simulink model "HIL_Testing_SW"  (Simulink 7.5)
settings: Solver=ode1  StartTime=0.0  StopTime=Inf  FixedStep=0.001  RelTol=1e-3
PostLoadFcn:
  | , if any(exist('dsrtsu_mdlpostloadfcn', 'file') == [2, 3, 6]), try dsrtsu_mdlpostloadfcn('Execute', bdroot); catch fprintf('Error in PostLoadFcn (dsrtsu_mdlpostloadfcn) for model "%s":\n %s\n', bdroot, lasterr); end, end,
undefined symbols (not defined in the file): CeBSER_Cnt_NumTempAxisPts, ChargeCord, ChargeCord_Control, ChargeToSOCCurr, ChrgCurrLim, CrntSens1Fine, CS_SOCSetPt, CyclerMaxChrgPwr, CyclerMaxDschrgPwr, deltaAhr, Drive_1, Drive_10, Drive_11, Drive_12, Drive_13, Drive_14, Drive_15, Drive_16, Drive_17, Drive_18, Drive_19, Drive_2, Drive_20, Drive_21, Drive_22, Drive_23, Drive_24, Drive_25, Drive_26, Drive_27, Drive_28, Drive_29, Drive_3, Drive_30, Drive_31, Drive_32, Drive_33, Drive_34, Drive_35, Drive_36, Drive_37, Drive_38, Drive_39, Drive_4, Drive_40, Drive_41, Drive_42, Drive_43, Drive_44, Drive_45, Drive_46, Drive_47, Drive_48, Drive_49, Drive_5, Drive_50, Drive_51, Drive_6, Drive_7, Drive_8 ... (+50)
libraries: simulink x129, rtican x50, rti2211sailib x5, rti2211serlib x5, rti2202miolib x3
(part 20 of 23)

== system HIL_Testing_SW/TX/Chiller/ChillerCmndTxDecision/ChillerRxProcessing/ReadChillerSP/RxReadChillerSP7Bytes ==
  Action Port : ActionPort  ActionType=then
  ASCIILUTable : Lookup  InputValues=[48,49,50,51,52,53,54,55,56,57]  Table=[0,1,2,3,4,5,6,7,8,9]  LookUpMeth=Use Input Nearest  OutDataTypeMode=single  OutDataType=fixdt(1, 16)  OutScaling=2^0  OutDataTypeStr=single  RndMeth=Nearest
  ASCIILUTable1 : Lookup  InputValues=[48,49,50,51,52,53,54,55,56,57]  Table=[0,1,2,3,4,5,6,7,8,9]  LookUpMeth=Use Input Nearest  OutDataTypeMode=single  OutDataType=fixdt(1, 16)  OutScaling=2^0  OutDataTypeStr=single  RndMeth=Nearest
  ASCIILUTable2 : Lookup  InputValues=[48,49,50,51,52,53,54,55,56,57]  Table=[0,.1,.2,.3,.4,.5,.6,.7,.8,.9]  LookUpMeth=Use Input Nearest  OutDataTypeMode=single  OutDataType=fixdt(1, 16)  OutScaling=2^0  OutDataTypeStr=single  RndMeth=Nearest
  Add : Sum  Inputs=+++  OutDataType=fixdt(1, 16)  OutScaling=2^-10
  Constant : Constant  Value=43  OutDataTypeMode=uint16  OutDataType=fixdt(1, 16)  OutScaling=2^0  OutDataTypeStr=uint16
  Constant1 : Constant  Value=10  OutDataTypeMode=single  OutDataType=fixdt(1, 16)  OutScaling=2^0  OutDataTypeStr=single
  Constant4 : Constant  Value=-1  OutDataTypeMode=single  OutDataType=fixdt(1, 16)  OutScaling=2^0  OutDataTypeStr=single
  Constant5 : Constant  OutDataTypeMode=single  OutDataType=fixdt(1, 16)  OutScaling=2^0  OutDataTypeStr=single
  Data Store Read1 : DataStoreRead  DataStoreName=RxChillerFIFO  SampleTime=-1
  Demux : Demux  Outputs=7
  Gain : Gain  ParameterDataType=fixdt(1, 16)  ParameterScaling=2^0  OutDataType=fixdt(1, 16)  OutScaling=2^0
  Product : Product  OutDataType=fixdt(1, 16)  OutScaling=2^0  RndMeth=Zero
  Product1 : Product  OutDataTypeMode=single  OutDataType=fixdt(1, 16)  OutScaling=2^0  OutDataTypeStr=single  RndMeth=Zero
  Relational Operator3 : RelationalOperator  Operator===  LogicOutDataTypeMode=boolean  LogicDataType=fixdt(0, 8)  OutDataTypeStr=boolean
  Switch : Switch  Threshold=1  OutDataType=fixdt(1, 16)  OutScaling=2^0
  Terminator2 : Terminator
  Terminator3 : Terminator
  Terminator4 : Terminator
  RxReadChillerSetPoint : Outport  OutDataType=fixdt(1, 16)  OutScaling=2^0
  wires:
  [RxByteOne] -> Relational Operator3/1
  Constant/1 -> Relational Operator3/2
  [RxByteFour] -> ASCIILUTable1/1
  Relational Operator3/1 -> Switch/2
  Constant5/1 -> Switch/1
  Constant4/1 -> Switch/3
  Switch/1 -> [Sign]
  Constant1/1 -> Product/2
  [RxByteThree] -> ASCIILUTable/1
  ASCIILUTable/1 -> Product/1
  Product/1 -> [TensNumber]
  ASCIILUTable1/1 -> [OnesNumber]
  [RxByteSix] -> ASCIILUTable2/1
  ASCIILUTable2/1 -> [TenthsNumber]
  [TensNumber] -> Add/1
  [OnesNumber] -> Add/2
  [TenthsNumber] -> Add/3
  Add/1 -> Product1/2  "AddedChillSP"
  Demux/1 -> [RxByteOne]
  Demux/2 -> Terminator2/1
  Demux/3 -> [RxByteThree]
  Demux/4 -> [RxByteFour]
  Demux/5 -> Terminator3/1
  Demux/6 -> [RxByteSix]
  Demux/7 -> Terminator4/1
  Data Store Read1/1 -> Demux/1
  [Sign] -> Product1/1
  Product1/1 -> Gain/1
  Gain/1 -> RxReadChillerSetPoint/1

== system HIL_Testing_SW/TX/Chiller/ChillerCmndTxDecision/ChillerRxProcessing/ReadChillerTemp/RxReadChillerTemp4Bytes ==
  Action Port : ActionPort  ActionType=elseif
  ASCIILUTable : Lookup  InputValues=[48,49,50,51,52,53,54,55,56,57]  Table=[0,1,2,3,4,5,6,7,8,9]  LookUpMeth=Use Input Nearest  OutDataTypeMode=single  OutDataType=fixdt(1, 16)  OutScaling=2^0  OutDataTypeStr=single  RndMeth=Nearest
  ASCIILUTable1 : Lookup  InputValues=[48,49,50,51,52,53,54,55,56,57]  Table=[0,1,2,3,4,5,6,7,8,9]  LookUpMeth=Use Input Nearest  OutDataTypeMode=single  OutDataType=fixdt(1, 16)  OutScaling=2^0  OutDataTypeStr=single  RndMeth=Nearest
  Add : Sum  Inputs=+++  OutDataType=fixdt(1, 16)  OutScaling=2^-10
  Constant : Constant  Value=43  OutDataTypeMode=uint16  OutDataType=fixdt(1, 16)  OutScaling=2^0  OutDataTypeStr=uint16
  Constant1 : Constant  Value=10  OutDataTypeMode=single  OutDataType=fixdt(1, 16)  OutScaling=2^0  OutDataTypeStr=single
  Constant2 : Constant  Value=0  OutDataTypeMode=single  OutDataType=fixdt(1, 16)  OutScaling=2^0  OutDataTypeStr=single
  Constant4 : Constant  Value=-1  OutDataTypeMode=single  OutDataType=fixdt(1, 16)  OutScaling=2^0  OutDataTypeStr=single
  Constant5 : Constant  OutDataTypeMode=single  OutDataType=fixdt(1, 16)  OutScaling=2^0  OutDataTypeStr=single
  Data Store Read1 : DataStoreRead  DataStoreName=RxChillerFIFO  SampleTime=-1
  Demux : Demux  Outputs=7
  Gain : Gain  ParameterDataType=fixdt(1, 16)  ParameterScaling=2^0  OutDataType=fixdt(1, 16)  OutScaling=2^0
  Product : Product  OutDataType=fixdt(1, 16)  OutScaling=2^0  RndMeth=Zero
  Product1 : Product  OutDataTypeMode=single  OutDataType=fixdt(1, 16)  OutScaling=2^0  OutDataTypeStr=single  RndMeth=Zero
  Relational Operator3 : RelationalOperator  Operator===  LogicOutDataTypeMode=boolean  LogicDataType=fixdt(0, 8)  OutDataTypeStr=boolean
  Switch : Switch  Threshold=1  OutDataType=fixdt(1, 16)  OutScaling=2^0
  Terminator{2..5} (4 alike) : Terminator
  RxReadChillerSetPoint : Outport  OutDataType=fixdt(1, 16)  OutScaling=2^0
  wires:
  [Sign] -> Product1/1
  Data Store Read1/1 -> Demux/1
  Demux/7 -> Terminator5/1
  Demux/6 -> Terminator4/1
  Demux/4 -> Terminator2/1
  Demux/3 -> [RxByteThree]
  Demux/2 -> [RxByteTwo]
  Demux/1 -> [RxByteOne]
  Add/1 -> Product1/2
  [TenthsNumber] -> Add/3
  [OnesNumber] -> Add/2
  [TensNumber] -> Add/1
  ASCIILUTable1/1 -> [OnesNumber]
  Product/1 -> [TensNumber]
  ASCIILUTable/1 -> Product/1
  [RxByteTwo] -> ASCIILUTable/1
  Constant1/1 -> Product/2
  Switch/1 -> [Sign]
  Constant4/1 -> Switch/3
  Constant5/1 -> Switch/1
  Relational Operator3/1 -> Switch/2
  [RxByteThree] -> ASCIILUTable1/1
  Constant/1 -> Relational Operator3/2
  [RxByteOne] -> Relational Operator3/1
  Constant2/1 -> [TenthsNumber]
  Demux/5 -> Terminator3/1
  Product1/1 -> Gain/1
  Gain/1 -> RxReadChillerSetPoint/1

== system HIL_Testing_SW/TX/Chiller/ChillerCmndTxDecision/ChillerRxProcessing/ReadChillerTemp/RxReadChillerTemp7Bytes ==
  Action Port : ActionPort  ActionType=then
  ASCIILUTable : Lookup  InputValues=[48,49,50,51,52,53,54,55,56,57]  Table=[0,1,2,3,4,5,6,7,8,9]  LookUpMeth=Use Input Nearest  OutDataTypeMode=single  OutDataType=fixdt(1, 16)  OutScaling=2^0  OutDataTypeStr=single  RndMeth=Nearest
  ASCIILUTable1 : Lookup  InputValues=[48,49,50,51,52,53,54,55,56,57]  Table=[0,1,2,3,4,5,6,7,8,9]  LookUpMeth=Use Input Nearest  OutDataTypeMode=single  OutDataType=fixdt(1, 16)  OutScaling=2^0  OutDataTypeStr=single  RndMeth=Nearest
  ASCIILUTable2 : Lookup  InputValues=[48,49,50,51,52,53,54,55,56,57]  Table=[0,.1,.2,.3,.4,.5,.6,.7,.8,.9]  LookUpMeth=Use Input Nearest  OutDataTypeMode=single  OutDataType=fixdt(1, 16)  OutScaling=2^0  OutDataTypeStr=single  RndMeth=Nearest
  Add : Sum  Inputs=+++  OutDataType=fixdt(1, 16)  OutScaling=2^-10
  Constant : Constant  Value=43  OutDataTypeMode=uint16  OutDataType=fixdt(1, 16)  OutScaling=2^0  OutDataTypeStr=uint16
  Constant1 : Constant  Value=10  OutDataTypeMode=single  OutDataType=fixdt(1, 16)  OutScaling=2^0  OutDataTypeStr=single
  Constant4 : Constant  Value=-1  OutDataTypeMode=single  OutDataType=fixdt(1, 16)  OutScaling=2^0  OutDataTypeStr=single
  Constant5 : Constant  OutDataTypeMode=single  OutDataType=fixdt(1, 16)  OutScaling=2^0  OutDataTypeStr=single
  Data Store Read1 : DataStoreRead  DataStoreName=RxChillerFIFO  SampleTime=-1
  Demux : Demux  Outputs=7
  Gain : Gain  ParameterDataType=fixdt(1, 16)  ParameterScaling=2^0  OutDataType=fixdt(1, 16)  OutScaling=2^0
  Product : Product  OutDataTypeMode=single  OutDataType=fixdt(1, 16)  OutScaling=2^0  OutDataTypeStr=single  RndMeth=Zero
  Product1 : Product  OutDataTypeMode=single  OutDataType=fixdt(1, 16)  OutScaling=2^0  OutDataTypeStr=single  RndMeth=Zero
  Relational Operator3 : RelationalOperator  Operator===  LogicOutDataTypeMode=boolean  LogicDataType=fixdt(0, 8)  OutDataTypeStr=boolean
  Switch : Switch  Threshold=1  OutDataTypeMode=single  OutDataType=fixdt(1, 16)  OutScaling=2^0  OutDataTypeStr=single
  Terminator2 : Terminator
  Terminator3 : Terminator
  Terminator4 : Terminator
  RxReadChillerSetPoint : Outport  OutDataType=fixdt(1, 16)  OutScaling=2^0
  wires:
  [RxByteOne] -> Relational Operator3/1
  Constant/1 -> Relational Operator3/2
  [RxByteFour] -> ASCIILUTable1/1
  Relational Operator3/1 -> Switch/2
  Constant5/1 -> Switch/1
  Constant4/1 -> Switch/3
  Switch/1 -> [Sign]
  Constant1/1 -> Product/2
  [RxByteThree] -> ASCIILUTable/1
  ASCIILUTable/1 -> Product/1
  Product/1 -> [TensNumber]
  ASCIILUTable1/1 -> [OnesNumber]
  [RxByteSix] -> ASCIILUTable2/1
  ASCIILUTable2/1 -> [TenthsNumber]
  [TensNumber] -> Add/1
  [OnesNumber] -> Add/2
  [TenthsNumber] -> Add/3
  Add/1 -> Product1/2  "AddedChillSP"
  [Sign] -> Product1/1
  Product1/1 -> Gain/1
  Demux/1 -> [RxByteOne]
  Demux/2 -> Terminator2/1
  Demux/3 -> [RxByteThree]
  Demux/4 -> [RxByteFour]
  Demux/5 -> Terminator3/1
  Demux/6 -> [RxByteSix]
  Demux/7 -> Terminator4/1
  Data Store Read1/1 -> Demux/1
  Gain/1 -> RxReadChillerSetPoint/1

== system HIL_Testing_SW/TX/Chiller/ChillerCmndTxDecision/ChillerRxProcessing/RxChillerByteShifter/NoShiftDaFIFO1 ==
  note: No Shift FIFO
  In1 : Inport  OutDataType=fixdt(1, 16)  OutScaling=2^0
  Action Port : ActionPort  ActionType=elseif
  Demux1 : Demux  Outputs=7
  Gain{,1..7} (8 alike) : Gain  ParameterDataType=fixdt(1, 16)  ParameterScaling=2^0  OutDataTypeMode=uint8  OutDataType=fixdt(1, 16)  OutScaling=2^0  OutDataTypeStr=uint8
  Mux : Mux  Inputs=7
  Out1 : Outport  OutDataType=fixdt(1, 16)  OutScaling=2^0
  wires:
  Mux/1 -> Gain7/1
  [RxByteOne] -> Mux/1
  [RxByteTwo] -> Mux/2
  [RxByteThree] -> Mux/3
  [RxByteFour] -> Mux/4
  [RxByteFive] -> Mux/5
  [RxByteSix] -> Mux/6
  [RxByteSeven] -> Mux/7
  Demux1/1 -> Gain/1
  Demux1/2 -> Gain1/1
  Demux1/3 -> Gain2/1
  Demux1/4 -> Gain3/1
  Demux1/5 -> Gain4/1
  Demux1/6 -> Gain5/1
  Demux1/7 -> Gain6/1
  Gain/1 -> [RxByteOne]
  Gain1/1 -> [RxByteTwo]
  Gain2/1 -> [RxByteThree]
  Gain3/1 -> [RxByteFour]
  Gain4/1 -> [RxByteFive]
  Gain5/1 -> [RxByteSix]
  Gain6/1 -> [RxByteSeven]
  In1/1 -> Demux1/1
  Gain7/1 -> Out1/1

== system HIL_Testing_SW/TX/Chiller/ChillerCmndTxDecision/ChillerRxProcessing/RxChillerByteShifter/NoShiftDaFIFO2 ==
  note: No Shift FIFO
  In1 : Inport  OutDataType=fixdt(1, 16)  OutScaling=2^0
  Action Port : ActionPort  ActionType=else
  Demux1 : Demux  Outputs=7
  Gain{,1..7} (8 alike) : Gain  ParameterDataType=fixdt(1, 16)  ParameterScaling=2^0  OutDataTypeMode=uint8  OutDataType=fixdt(1, 16)  OutScaling=2^0  OutDataTypeStr=uint8
  Mux : Mux  Inputs=7
  Out1 : Outport  OutDataType=fixdt(1, 16)  OutScaling=2^0
  wires:
  Gain7/1 -> Out1/1
  In1/1 -> Demux1/1
  Gain6/1 -> [RxByteSeven]
  Gain5/1 -> [RxByteSix]
  Gain4/1 -> [RxByteFive]
  Gain3/1 -> [RxByteFour]
  Gain2/1 -> [RxByteThree]
  Gain1/1 -> [RxByteTwo]
  Gain/1 -> [RxByteOne]
  Demux1/7 -> Gain6/1
  Demux1/6 -> Gain5/1
  Demux1/5 -> Gain4/1
  Demux1/4 -> Gain3/1
  Demux1/3 -> Gain2/1
  Demux1/2 -> Gain1/1
  Demux1/1 -> Gain/1
  [RxByteSeven] -> Mux/7
  [RxByteSix] -> Mux/6
  [RxByteFive] -> Mux/5
  [RxByteFour] -> Mux/4
  [RxByteThree] -> Mux/3
  [RxByteTwo] -> Mux/2
  [RxByteOne] -> Mux/1
  Mux/1 -> Gain7/1

== system HIL_Testing_SW/TX/Chiller/ChillerCmndTxDecision/ChillerRxProcessing/RxChillerByteShifter/PositiveResponseNoShift ==
  note: No Shift FIFO Right
  In1 : Inport  OutDataType=fixdt(1, 16)  OutScaling=2^0
  Action Port : ActionPort  ActionType=then
  Demux1 : Demux  Outputs=7
  Gain{,1..7} (8 alike) : Gain  ParameterDataType=fixdt(1, 16)  ParameterScaling=2^0  OutDataTypeMode=uint8  OutDataType=fixdt(1, 16)  OutScaling=2^0  OutDataTypeStr=uint8
  Mux : Mux  Inputs=7
  Out1 : Outport  OutDataType=fixdt(1, 16)  OutScaling=2^0
  wires:
  Mux/1 -> Gain7/1
  Demux1/1 -> Gain/1
  Demux1/2 -> Gain1/1
  Demux1/3 -> Gain2/1
  Demux1/4 -> Gain3/1
  Demux1/5 -> Gain4/1
  Demux1/6 -> Gain5/1
  Demux1/7 -> Gain6/1
  Gain/1 -> [RxByteOne]
  Gain1/1 -> [RxByteTwo]
  Gain2/1 -> [RxByteThree]
  Gain3/1 -> [RxByteFour]
  Gain4/1 -> [RxByteFive]
  Gain5/1 -> [RxByteSix]
  Gain6/1 -> [RxByteSeven]
  In1/1 -> Demux1/1
  Gain7/1 -> Out1/1
  [RxByteSeven] -> Mux/7
  [RxByteSix] -> Mux/6
  [RxByteFive] -> Mux/5
  [RxByteFour] -> Mux/4
  [RxByteThree] -> Mux/3
  [RxByteTwo] -> Mux/2
  [RxByteOne] -> Mux/1

== system HIL_Testing_SW/TX/Chiller/ChillerCmndTxDecision/ChillerRxProcessing/RxChillerByteShifter/ShiftFIFO_FiveRight ==
  note: Shift FIFO Five Right
  In1 : Inport  OutDataType=fixdt(1, 16)  OutScaling=2^0
  Action Port : ActionPort  ActionType=elseif
  Demux : Demux  Outputs=7
  Gain{,1..7} (8 alike) : Gain  ParameterDataType=fixdt(1, 16)  ParameterScaling=2^0  OutDataTypeMode=uint8  OutDataType=fixdt(1, 16)  OutScaling=2^0  OutDataTypeStr=uint8
  Mux : Mux  Inputs=7
  Out1 : Outport  OutDataType=fixdt(1, 16)  OutScaling=2^0
  wires:
  Mux/1 -> Gain7/1
  Demux/1 -> Gain/1
  Demux/2 -> Gain1/1
  Demux/3 -> Gain2/1
  Demux/4 -> Gain3/1
  Demux/5 -> Gain4/1
  Demux/6 -> Gain5/1
  Demux/7 -> Gain6/1
  In1/1 -> Demux/1
  Gain/1 -> [RxByteOne]
  Gain1/1 -> [RxByteTwo]
  Gain2/1 -> [RxByteThree]
  Gain3/1 -> [RxByteFour]
  Gain4/1 -> [RxByteFive]
  Gain5/1 -> [RxByteSix]
  Gain6/1 -> [RxByteSeven]
  Gain7/1 -> Out1/1
  [RxByteOne] -> Mux/6
  [RxByteSeven] -> Mux/5
  [RxByteSix] -> Mux/4
  [RxByteFive] -> Mux/3
  [RxByteFour] -> Mux/2
  [RxByteThree] -> Mux/1
  [RxByteTwo] -> Mux/7

== system HIL_Testing_SW/TX/Chiller/ChillerCmndTxDecision/ChillerRxProcessing/RxChillerByteShifter/ShiftFIFO_FourRight ==
  note: Shift FIFO Four Right
  In1 : Inport  OutDataType=fixdt(1, 16)  OutScaling=2^0
  Action Port : ActionPort  ActionType=elseif
  Demux1 : Demux  Outputs=7
  Gain{,1..7} (8 alike) : Gain  ParameterDataType=fixdt(1, 16)  ParameterScaling=2^0  OutDataTypeMode=uint8  OutDataType=fixdt(1, 16)  OutScaling=2^0  OutDataTypeStr=uint8
  Mux : Mux  Inputs=7
  Out1 : Outport  OutDataType=fixdt(1, 16)  OutScaling=2^0
  wires:
  Mux/1 -> Gain7/1
  [RxByteThree] -> Mux/7
  [RxByteTwo] -> Mux/6
  [RxByteOne] -> Mux/5
  [RxByteSeven] -> Mux/4
  [RxByteSix] -> Mux/3
  [RxByteFour] -> Mux/1
  [RxByteFive] -> Mux/2
  Demux1/1 -> Gain/1
  Demux1/2 -> Gain1/1
  Demux1/3 -> Gain2/1
  Demux1/4 -> Gain3/1
  Demux1/5 -> Gain4/1
  Demux1/6 -> Gain5/1
  Demux1/7 -> Gain6/1
  Gain/1 -> [RxByteOne]
  Gain1/1 -> [RxByteTwo]
  Gain2/1 -> [RxByteThree]
  Gain3/1 -> [RxByteFour]
  Gain4/1 -> [RxByteFive]
  Gain5/1 -> [RxByteSix]
  Gain6/1 -> [RxByteSeven]
  In1/1 -> Demux1/1
  Gain7/1 -> Out1/1

== system HIL_Testing_SW/TX/Chiller/ChillerCmndTxDecision/ChillerRxProcessing/RxChillerByteShifter/ShiftFIFO_OneRight ==
  note: Shift FIFO One Right
  In1 : Inport  OutDataType=fixdt(1, 16)  OutScaling=2^0
  Action Port : ActionPort  ActionType=elseif
  Demux1 : Demux  Outputs=7
  Gain{,1..7} (8 alike) : Gain  ParameterDataType=fixdt(1, 16)  ParameterScaling=2^0  OutDataTypeMode=uint8  OutDataType=fixdt(1, 16)  OutScaling=2^0  OutDataTypeStr=uint8
  Mux : Mux  Inputs=7
  Out1 : Outport  OutDataType=fixdt(1, 16)  OutScaling=2^0
  wires:
  Mux/1 -> Gain7/1
  Demux1/1 -> Gain/1
  Demux1/2 -> Gain1/1
  Demux1/3 -> Gain2/1
  Demux1/4 -> Gain3/1
  Demux1/5 -> Gain4/1
  Demux1/6 -> Gain5/1
  Demux1/7 -> Gain6/1
  Gain/1 -> [RxByteOne]
  Gain1/1 -> [RxByteTwo]
  Gain2/1 -> [RxByteThree]
  Gain3/1 -> [RxByteFour]
  Gain4/1 -> [RxByteFive]
  Gain5/1 -> [RxByteSix]
  Gain6/1 -> [RxByteSeven]
  In1/1 -> Demux1/1
  Gain7/1 -> Out1/1
  [RxByteTwo] -> Mux/3
  [RxByteThree] -> Mux/4
  [RxByteFour] -> Mux/5
  [RxByteFive] -> Mux/6
  [RxByteSix] -> Mux/7
  [RxByteOne] -> Mux/2
  [RxByteSeven] -> Mux/1

== system HIL_Testing_SW/TX/Chiller/ChillerCmndTxDecision/ChillerRxProcessing/RxChillerByteShifter/ShiftFIFO_SixRight ==
  note: Shift FIFO Six Right
  In1 : Inport  OutDataType=fixdt(1, 16)  OutScaling=2^0
  Action Port : ActionPort  ActionType=elseif
  Demux : Demux  Outputs=7
  Gain{,1..7} (8 alike) : Gain  ParameterDataType=fixdt(1, 16)  ParameterScaling=2^0  OutDataTypeMode=uint8  OutDataType=fixdt(1, 16)  OutScaling=2^0  OutDataTypeStr=uint8
  Mux : Mux  Inputs=7
  Out1 : Outport  OutDataType=fixdt(1, 16)  OutScaling=2^0
  wires:
  Demux/1 -> Gain/1
  Demux/2 -> Gain1/1
  Demux/3 -> Gain2/1
  Demux/4 -> Gain3/1
  Demux/5 -> Gain4/1
  Demux/6 -> Gain5/1
  Demux/7 -> Gain6/1
  In1/1 -> Demux/1
  Mux/1 -> Gain7/1
  Gain6/1 -> [RxByteSeven]
  Gain5/1 -> [RxByteSix]
  Gain4/1 -> [RxByteFive]
  Gain3/1 -> [RxByteFour]
  Gain2/1 -> [RxByteThree]
  Gain1/1 -> [RxByteTwo]
  Gain/1 -> [RxByteOne]
  Gain7/1 -> Out1/1
  [RxByteOne] -> Mux/7
  [RxByteSeven] -> Mux/6
  [RxByteSix] -> Mux/5
  [RxByteFive] -> Mux/4
  [RxByteFour] -> Mux/3
  [RxByteThree] -> Mux/2
  [RxByteTwo] -> Mux/1

== system HIL_Testing_SW/TX/Chiller/ChillerCmndTxDecision/ChillerRxProcessing/RxChillerByteShifter/ShiftFIFO_ThreeRight ==
  note: Shift FIFO Three Right
  In2 : Inport  OutDataType=fixdt(1, 16)  OutScaling=2^0
  Action Port : ActionPort  ActionType=elseif
  Demux2 : Demux  Outputs=7
  Gain{8..15} (8 alike) : Gain  ParameterDataType=fixdt(1, 16)  ParameterScaling=2^0  OutDataTypeMode=uint8  OutDataType=fixdt(1, 16)  OutScaling=2^0  OutDataTypeStr=uint8
  Mux1 : Mux  Inputs=7
  Out2 : Outport  OutDataType=fixdt(1, 16)  OutScaling=2^0
  wires:
  Mux1/1 -> Gain15/1
  [RxByteSix] -> Mux1/2
  [RxByteSeven] -> Mux1/3
  [RxByteOne] -> Mux1/4
  [RxByteTwo] -> Mux1/5
  [RxByteThree] -> Mux1/6
  [RxByteFour] -> Mux1/7
  [RxByteFive] -> Mux1/1
  Demux2/1 -> Gain8/1
  Demux2/2 -> Gain9/1
  Demux2/3 -> Gain10/1
  Demux2/4 -> Gain11/1
  Demux2/5 -> Gain12/1
  Demux2/6 -> Gain13/1
  Demux2/7 -> Gain14/1
  Gain8/1 -> [RxByteOne]
  Gain9/1 -> [RxByteTwo]
  Gain10/1 -> [RxByteThree]
  Gain11/1 -> [RxByteFour]
  Gain12/1 -> [RxByteFive]
  Gain13/1 -> [RxByteSix]
  Gain14/1 -> [RxByteSeven]
  In2/1 -> Demux2/1
  Gain15/1 -> Out2/1

== system HIL_Testing_SW/TX/Chiller/ChillerCmndTxDecision/ChillerRxProcessing/RxChillerByteShifter/ShiftFIFO_TwoRight ==
  note: Shift FIFO Two Right
  In1 : Inport  OutDataType=fixdt(1, 16)  OutScaling=2^0
  Action Port : ActionPort  ActionType=elseif
  Demux : Demux  Outputs=7
  Gain{,1..7} (8 alike) : Gain  ParameterDataType=fixdt(1, 16)  ParameterScaling=2^0  OutDataTypeMode=uint8  OutDataType=fixdt(1, 16)  OutScaling=2^0  OutDataTypeStr=uint8
  Mux : Mux  Inputs=7
  Out1 : Outport  OutDataType=fixdt(1, 16)  OutScaling=2^0
  wires:
  Mux/1 -> Gain7/1
  [RxByteSeven] -> Mux/2
  [RxByteOne] -> Mux/3
  [RxByteTwo] -> Mux/4
  [RxByteThree] -> Mux/5
  [RxByteFour] -> Mux/6
  [RxByteFive] -> Mux/7
  [RxByteSix] -> Mux/1
  Demux/1 -> Gain/1
  Demux/2 -> Gain1/1
  Demux/3 -> Gain2/1
  Demux/4 -> Gain3/1
  Demux/5 -> Gain4/1
  Demux/6 -> Gain5/1
  Demux/7 -> Gain6/1
  In1/1 -> Demux/1
  Gain/1 -> [RxByteOne]
  Gain1/1 -> [RxByteTwo]
  Gain2/1 -> [RxByteThree]
  Gain3/1 -> [RxByteFour]
  Gain4/1 -> [RxByteFive]
  Gain5/1 -> [RxByteSix]
  Gain6/1 -> [RxByteSeven]
  Gain7/1 -> Out1/1

== system HIL_Testing_SW/TX/Chiller/ChillerCmndTxDecision/ChillerRxProcessing/RxChillerByteShifter/SwapByte1And2 ==
  note: SwapByte1And2
  In1 : Inport  OutDataType=fixdt(1, 16)  OutScaling=2^0
  Action Port : ActionPort  ActionType=elseif
  Demux1 : Demux  Outputs=7
  Gain{,1..7} (8 alike) : Gain  ParameterDataType=fixdt(1, 16)  ParameterScaling=2^0  OutDataTypeMode=uint8  OutDataType=fixdt(1, 16)  OutScaling=2^0  OutDataTypeStr=uint8
  Mux : Mux  Inputs=7
  Out1 : Outport  OutDataType=fixdt(1, 16)  OutScaling=2^0
  wires:
  [RxByteThree] -> Mux/3
  [RxByteFour] -> Mux/4
  [RxByteFive] -> Mux/5
  [RxByteSix] -> Mux/6
  [RxByteSeven] -> Mux/7
  Gain7/1 -> Out1/1
  In1/1 -> Demux1/1
  Gain6/1 -> [RxByteSeven]
  Gain5/1 -> [RxByteSix]
  Gain4/1 -> [RxByteFive]
  Gain3/1 -> [RxByteFour]
  Gain2/1 -> [RxByteThree]
  Gain1/1 -> [RxByteTwo]
  Gain/1 -> [RxByteOne]
  Demux1/7 -> Gain6/1
  Demux1/6 -> Gain5/1
  Demux1/5 -> Gain4/1
  Demux1/4 -> Gain3/1
  Demux1/3 -> Gain2/1
  Demux1/2 -> Gain1/1
  Demux1/1 -> Gain/1
  Mux/1 -> Gain7/1
  [RxByteTwo] -> Mux/1
  [RxByteOne] -> Mux/2

== system HIL_Testing_SW/LionsHeart/FeaturePresentation/Down_to_Business/DriveProfile_ModeControl/Drive_Profile/CD/Drive 1 ==
  loop_time : Inport  OutDataType=sfix(16)  OutScaling=2^0
  Enable : EnablePort
  Lookup Table : Lookup  InputValues=Drive_1(:,1)  Table=Drive_1(:,2)  OutDataType=fixdt(1, 16)  OutScaling=2^0
  Product1 : Product  OutDataType=sfix(16)  OutScaling=2^0  RndMeth=Zero
  W_kW : Constant  Value=single(1000)  OutDataType=sfix(16)  OutScaling=2^0
  Profile_Data : Outport  OutDataType=sfix(16)  OutScaling=2^0
  wires:
  Product1/1 -> Profile_Data/1
  Lookup Table/1 -> Product1/1
  W_kW/1 -> Product1/2
  loop_time/1 -> Lookup Table/1

== system HIL_Testing_SW/LionsHeart/FeaturePresentation/Down_to_Business/DriveProfile_ModeControl/Drive_Profile/CD/Drive 2 ==
  loop_time : Inport  OutDataType=sfix(16)  OutScaling=2^0
  Enable : EnablePort
  Lookup Table : Lookup  InputValues=Drive_2(:,1)  Table=Drive_2(:,2)  OutDataType=fixdt(1, 16)  OutScaling=2^0
  Product1 : Product  OutDataType=sfix(16)  OutScaling=2^0  RndMeth=Zero
  W_kW : Constant  Value=single(1000)  OutDataType=sfix(16)  OutScaling=2^0
  Profile_Data : Outport  OutDataType=sfix(16)  OutScaling=2^0
  wires:
  Product1/1 -> Profile_Data/1
  Lookup Table/1 -> Product1/1
  W_kW/1 -> Product1/2
  loop_time/1 -> Lookup Table/1

== system HIL_Testing_SW/LionsHeart/FeaturePresentation/Down_to_Business/DriveProfile_ModeControl/Drive_Profile/CD/Drive_10 ==
  loop_time : Inport  OutDataType=sfix(16)  OutScaling=2^0
  Enable : EnablePort
  Lookup Table : Lookup  InputValues=Drive_10(:,1)  Table=Drive_10(:,2)  OutDataType=fixdt(1, 16)  OutScaling=2^0
  Product1 : Product  OutDataType=sfix(16)  OutScaling=2^0  RndMeth=Zero
  W_kW : Constant  Value=single(1000)  OutDataType=sfix(16)  OutScaling=2^0
  Profile_Data : Outport  OutDataType=sfix(16)  OutScaling=2^0
  wires:
  Product1/1 -> Profile_Data/1
  Lookup Table/1 -> Product1/1
  W_kW/1 -> Product1/2
  loop_time/1 -> Lookup Table/1

== system HIL_Testing_SW/LionsHeart/FeaturePresentation/Down_to_Business/DriveProfile_ModeControl/Drive_Profile/CD/Drive_11 ==
  loop_time : Inport  OutDataType=sfix(16)  OutScaling=2^0
  Enable : EnablePort
  Lookup Table : Lookup  InputValues=Drive_11(:,1)  Table=Drive_11(:,2)  OutDataType=fixdt(1, 16)  OutScaling=2^0
  Product1 : Product  OutDataType=sfix(16)  OutScaling=2^0  RndMeth=Zero
  W_kW : Constant  Value=single(1000)  OutDataType=sfix(16)  OutScaling=2^0
  Profile_Data : Outport  OutDataType=sfix(16)  OutScaling=2^0
  wires:
  loop_time/1 -> Lookup Table/1
  W_kW/1 -> Product1/2
  Lookup Table/1 -> Product1/1
  Product1/1 -> Profile_Data/1

== system HIL_Testing_SW/LionsHeart/FeaturePresentation/Down_to_Business/DriveProfile_ModeControl/Drive_Profile/CD/Drive_12 ==
  loop_time : Inport  OutDataType=sfix(16)  OutScaling=2^0
  Enable : EnablePort
  Lookup Table : Lookup  InputValues=Drive_12(:,1)  Table=Drive_12(:,2)  OutDataType=fixdt(1, 16)  OutScaling=2^0
  Product1 : Product  OutDataType=sfix(16)  OutScaling=2^0  RndMeth=Zero
  W_kW : Constant  Value=single(1000)  OutDataType=sfix(16)  OutScaling=2^0
  Profile_Data : Outport  OutDataType=sfix(16)  OutScaling=2^0
  wires:
  Product1/1 -> Profile_Data/1
  Lookup Table/1 -> Product1/1
  W_kW/1 -> Product1/2
  loop_time/1 -> Lookup Table/1

== system HIL_Testing_SW/LionsHeart/FeaturePresentation/Down_to_Business/DriveProfile_ModeControl/Drive_Profile/CD/Drive_13 ==
  loop_time : Inport  OutDataType=sfix(16)  OutScaling=2^0
  Enable : EnablePort
  Lookup Table : Lookup  InputValues=Drive_13(:,1)  Table=Drive_13(:,2)  OutDataType=fixdt(1, 16)  OutScaling=2^0
  Product1 : Product  OutDataType=sfix(16)  OutScaling=2^0  RndMeth=Zero
  W_kW : Constant  Value=single(1000)  OutDataType=sfix(16)  OutScaling=2^0
  Profile_Data : Outport  OutDataType=sfix(16)  OutScaling=2^0
  wires:
  Product1/1 -> Profile_Data/1
  Lookup Table/1 -> Product1/1
  W_kW/1 -> Product1/2
  loop_time/1 -> Lookup Table/1

== system HIL_Testing_SW/LionsHeart/FeaturePresentation/Down_to_Business/DriveProfile_ModeControl/Drive_Profile/CD/Drive_14 ==
  loop_time : Inport  OutDataType=sfix(16)  OutScaling=2^0
  Enable : EnablePort
  Lookup Table : Lookup  InputValues=Drive_14(:,1)  Table=Drive_14(:,2)  OutDataType=fixdt(1, 16)  OutScaling=2^0
  Product1 : Product  OutDataType=sfix(16)  OutScaling=2^0  RndMeth=Zero
  W_kW : Constant  Value=single(1000)  OutDataType=sfix(16)  OutScaling=2^0
  Profile_Data : Outport  OutDataType=sfix(16)  OutScaling=2^0
  wires:
  Product1/1 -> Profile_Data/1
  Lookup Table/1 -> Product1/1
  W_kW/1 -> Product1/2
  loop_time/1 -> Lookup Table/1

== system HIL_Testing_SW/LionsHeart/FeaturePresentation/Down_to_Business/DriveProfile_ModeControl/Drive_Profile/CD/Drive_15 ==
  loop_time : Inport  OutDataType=sfix(16)  OutScaling=2^0
  Enable : EnablePort
  Lookup Table : Lookup  InputValues=Drive_15(:,1)  Table=Drive_15(:,2)  OutDataType=fixdt(1, 16)  OutScaling=2^0
  Product1 : Product  OutDataType=sfix(16)  OutScaling=2^0  RndMeth=Zero
  W_kW : Constant  Value=single(1000)  OutDataType=sfix(16)  OutScaling=2^0
  Profile_Data : Outport  OutDataType=sfix(16)  OutScaling=2^0
  wires:
  Product1/1 -> Profile_Data/1
  Lookup Table/1 -> Product1/1
  W_kW/1 -> Product1/2
  loop_time/1 -> Lookup Table/1

== system HIL_Testing_SW/LionsHeart/FeaturePresentation/Down_to_Business/DriveProfile_ModeControl/Drive_Profile/CD/Drive_16 ==
  loop_time : Inport  OutDataType=sfix(16)  OutScaling=2^0
  Enable : EnablePort
  Lookup Table : Lookup  InputValues=Drive_16(:,1)  Table=Drive_16(:,2)  OutDataType=fixdt(1, 16)  OutScaling=2^0
  Product1 : Product  OutDataType=sfix(16)  OutScaling=2^0  RndMeth=Zero
  W_kW : Constant  Value=single(1000)  OutDataType=sfix(16)  OutScaling=2^0
  Profile_Data : Outport  OutDataType=sfix(16)  OutScaling=2^0
  wires:
  Product1/1 -> Profile_Data/1
  Lookup Table/1 -> Product1/1
  W_kW/1 -> Product1/2
  loop_time/1 -> Lookup Table/1

== system HIL_Testing_SW/LionsHeart/FeaturePresentation/Down_to_Business/DriveProfile_ModeControl/Drive_Profile/CD/Drive_17 ==
  loop_time : Inport  OutDataType=sfix(16)  OutScaling=2^0
  Enable : EnablePort
  Lookup Table : Lookup  InputValues=Drive_17(:,1)  Table=Drive_17(:,2)  OutDataType=fixdt(1, 16)  OutScaling=2^0
  Product1 : Product  OutDataType=sfix(16)  OutScaling=2^0  RndMeth=Zero
  W_kW : Constant  Value=single(1000)  OutDataType=sfix(16)  OutScaling=2^0
  Profile_Data : Outport  OutDataType=sfix(16)  OutScaling=2^0
  wires:
  Product1/1 -> Profile_Data/1
  Lookup Table/1 -> Product1/1
  W_kW/1 -> Product1/2
  loop_time/1 -> Lookup Table/1

== system HIL_Testing_SW/LionsHeart/FeaturePresentation/Down_to_Business/DriveProfile_ModeControl/Drive_Profile/CD/Drive_18 ==
  loop_time : Inport  OutDataType=sfix(16)  OutScaling=2^0
  Enable : EnablePort
  Lookup Table : Lookup  InputValues=Drive_18(:,1)  Table=Drive_18(:,2)  OutDataType=fixdt(1, 16)  OutScaling=2^0
  Product2 : Product  OutDataType=sfix(16)  OutScaling=2^0  RndMeth=Zero
  W_kW1 : Constant  Value=single(1000)  OutDataType=sfix(16)  OutScaling=2^0
  Profile_Data : Outport  OutDataType=sfix(16)  OutScaling=2^0
  wires:
  loop_time/1 -> Lookup Table/1
  W_kW1/1 -> Product2/2
  Lookup Table/1 -> Product2/1
  Product2/1 -> Profile_Data/1

== system HIL_Testing_SW/LionsHeart/FeaturePresentation/Down_to_Business/DriveProfile_ModeControl/Drive_Profile/CD/Drive_19 ==
  loop_time : Inport  OutDataType=sfix(16)  OutScaling=2^0
  Enable : EnablePort
  Lookup Table : Lookup  InputValues=Drive_19(:,1)  Table=Drive_19(:,2)  OutDataType=fixdt(1, 16)  OutScaling=2^0
  Product2 : Product  OutDataType=sfix(16)  OutScaling=2^0  RndMeth=Zero
  W_kW1 : Constant  Value=single(1000)  OutDataType=sfix(16)  OutScaling=2^0
  Profile_Data : Outport  OutDataType=sfix(16)  OutScaling=2^0
  wires:
  loop_time/1 -> Lookup Table/1
  W_kW1/1 -> Product2/2
  Lookup Table/1 -> Product2/1
  Product2/1 -> Profile_Data/1

== system HIL_Testing_SW/LionsHeart/FeaturePresentation/Down_to_Business/DriveProfile_ModeControl/Drive_Profile/CD/Drive_20 ==
  loop_time : Inport  OutDataType=sfix(16)  OutScaling=2^0
  Enable : EnablePort
  Lookup Table : Lookup  InputValues=Drive_20(:,1)  Table=Drive_20(:,2)  OutDataType=fixdt(1, 16)  OutScaling=2^0
  Product2 : Product  OutDataType=sfix(16)  OutScaling=2^0  RndMeth=Zero
  W_kW1 : Constant  Value=single(1000)  OutDataType=sfix(16)  OutScaling=2^0
  Profile_Data : Outport  OutDataType=sfix(16)  OutScaling=2^0
  wires:
  W_kW1/1 -> Product2/2
  Lookup Table/1 -> Product2/1
  Product2/1 -> Profile_Data/1
  loop_time/1 -> Lookup Table/1

== system HIL_Testing_SW/LionsHeart/FeaturePresentation/Down_to_Business/DriveProfile_ModeControl/Drive_Profile/CD/Drive_21 ==
  loop_time : Inport  OutDataType=sfix(16)  OutScaling=2^0
  Enable : EnablePort
  Lookup Table : Lookup  InputValues=Drive_21(:,1)  Table=Drive_21(:,2)  OutDataType=fixdt(1, 16)  OutScaling=2^0
  Product1 : Product  OutDataType=sfix(16)  OutScaling=2^0  RndMeth=Zero
  W_kW : Constant  Value=single(1000)  OutDataType=sfix(16)  OutScaling=2^0
  Profile_Data : Outport  OutDataType=sfix(16)  OutScaling=2^0
  wires:
  Product1/1 -> Profile_Data/1
  Lookup Table/1 -> Product1/1
  W_kW/1 -> Product1/2
  loop_time/1 -> Lookup Table/1

== system HIL_Testing_SW/LionsHeart/FeaturePresentation/Down_to_Business/DriveProfile_ModeControl/Drive_Profile/CD/Drive_22 ==
  loop_time : Inport  OutDataType=sfix(16)  OutScaling=2^0
  Enable : EnablePort
  Lookup Table : Lookup  InputValues=Drive_22(:,1)  Table=Drive_22(:,2)  OutDataType=fixdt(1, 16)  OutScaling=2^0
  Product1 : Product  OutDataType=sfix(16)  OutScaling=2^0  RndMeth=Zero
  W_kW : Constant  Value=single(1000)  OutDataType=sfix(16)  OutScaling=2^0
  Profile_Data : Outport  OutDataType=sfix(16)  OutScaling=2^0
  wires:
  loop_time/1 -> Lookup Table/1
  W_kW/1 -> Product1/2
  Lookup Table/1 -> Product1/1
  Product1/1 -> Profile_Data/1

== system HIL_Testing_SW/LionsHeart/FeaturePresentation/Down_to_Business/DriveProfile_ModeControl/Drive_Profile/CD/Drive_23 ==
  loop_time : Inport  OutDataType=sfix(16)  OutScaling=2^0
  Enable : EnablePort
  Lookup Table : Lookup  InputValues=Drive_23(:,1)  Table=Drive_23(:,2)  OutDataType=fixdt(1, 16)  OutScaling=2^0
  Product1 : Product  OutDataType=sfix(16)  OutScaling=2^0  RndMeth=Zero
  W_kW : Constant  Value=single(1000)  OutDataType=sfix(16)  OutScaling=2^0
  Profile_Data : Outport  OutDataType=sfix(16)  OutScaling=2^0
  wires:
  Product1/1 -> Profile_Data/1
  Lookup Table/1 -> Product1/1
  W_kW/1 -> Product1/2
  loop_time/1 -> Lookup Table/1

== system HIL_Testing_SW/LionsHeart/FeaturePresentation/Down_to_Business/DriveProfile_ModeControl/Drive_Profile/CD/Drive_24 ==
  loop_time : Inport  OutDataType=sfix(16)  OutScaling=2^0
  Enable : EnablePort
  Lookup Table : Lookup  InputValues=Drive_24(:,1)  Table=Drive_24(:,2)  OutDataType=fixdt(1, 16)  OutScaling=2^0
  Product1 : Product  OutDataType=sfix(16)  OutScaling=2^0  RndMeth=Zero
  W_kW : Constant  Value=single(1000)  OutDataType=sfix(16)  OutScaling=2^0
  Profile_Data : Outport  OutDataType=sfix(16)  OutScaling=2^0
  wires:
  Product1/1 -> Profile_Data/1
  Lookup Table/1 -> Product1/1
  W_kW/1 -> Product1/2
  loop_time/1 -> Lookup Table/1

== system HIL_Testing_SW/LionsHeart/FeaturePresentation/Down_to_Business/DriveProfile_ModeControl/Drive_Profile/CD/Drive_25 ==
  loop_time : Inport  OutDataType=sfix(16)  OutScaling=2^0
  Enable : EnablePort
  Lookup Table : Lookup  InputValues=Drive_25(:,1)  Table=Drive_25(:,2)  OutDataType=fixdt(1, 16)  OutScaling=2^0
  Product1 : Product  OutDataType=sfix(16)  OutScaling=2^0  RndMeth=Zero
  W_kW : Constant  Value=single(1000)  OutDataType=sfix(16)  OutScaling=2^0
  Profile_Data : Outport  OutDataType=sfix(16)  OutScaling=2^0
  wires:
  Product1/1 -> Profile_Data/1
  Lookup Table/1 -> Product1/1
  W_kW/1 -> Product1/2
  loop_time/1 -> Lookup Table/1

== system HIL_Testing_SW/LionsHeart/FeaturePresentation/Down_to_Business/DriveProfile_ModeControl/Drive_Profile/CD/Drive_26 ==
  loop_time : Inport  OutDataType=sfix(16)  OutScaling=2^0
  Enable : EnablePort
  Lookup Table : Lookup  InputValues=Drive_26(:,1)  Table=Drive_26(:,2)  OutDataType=fixdt(1, 16)  OutScaling=2^0
  Product1 : Product  OutDataType=sfix(16)  OutScaling=2^0  RndMeth=Zero
  W_kW : Constant  Value=single(1000)  OutDataType=sfix(16)  OutScaling=2^0
  Profile_Data : Outport  OutDataType=sfix(16)  OutScaling=2^0
  wires:
  Product1/1 -> Profile_Data/1
  Lookup Table/1 -> Product1/1
  W_kW/1 -> Product1/2
  loop_time/1 -> Lookup Table/1

== system HIL_Testing_SW/LionsHeart/FeaturePresentation/Down_to_Business/DriveProfile_ModeControl/Drive_Profile/CD/Drive_27 ==
  loop_time : Inport  OutDataType=sfix(16)  OutScaling=2^0
  Enable : EnablePort
  Lookup Table : Lookup  InputValues=Drive_27(:,1)  Table=Drive_27(:,2)  OutDataType=fixdt(1, 16)  OutScaling=2^0
  Product1 : Product  OutDataType=sfix(16)  OutScaling=2^0  RndMeth=Zero
  W_kW : Constant  Value=single(1000)  OutDataType=sfix(16)  OutScaling=2^0
  Profile_Data : Outport  OutDataType=sfix(16)  OutScaling=2^0
  wires:
  loop_time/1 -> Lookup Table/1
  W_kW/1 -> Product1/2
  Lookup Table/1 -> Product1/1
  Product1/1 -> Profile_Data/1

== system HIL_Testing_SW/LionsHeart/FeaturePresentation/Down_to_Business/DriveProfile_ModeControl/Drive_Profile/CD/Drive_28 ==
  loop_time : Inport  OutDataType=sfix(16)  OutScaling=2^0
  Enable : EnablePort
  Lookup Table : Lookup  InputValues=Drive_28(:,1)  Table=Drive_28(:,2)  OutDataType=fixdt(1, 16)  OutScaling=2^0
  Product1 : Product  OutDataType=sfix(16)  OutScaling=2^0  RndMeth=Zero
  W_kW : Constant  Value=single(1000)  OutDataType=sfix(16)  OutScaling=2^0
  Profile_Data : Outport  OutDataType=sfix(16)  OutScaling=2^0
  wires:
  Product1/1 -> Profile_Data/1
  Lookup Table/1 -> Product1/1
  W_kW/1 -> Product1/2
  loop_time/1 -> Lookup Table/1

== system HIL_Testing_SW/LionsHeart/FeaturePresentation/Down_to_Business/DriveProfile_ModeControl/Drive_Profile/CD/Drive_29 ==
  loop_time : Inport  OutDataType=sfix(16)  OutScaling=2^0
  Enable : EnablePort
  Lookup Table : Lookup  InputValues=Drive_29(:,1)  Table=Drive_29(:,2)  OutDataType=fixdt(1, 16)  OutScaling=2^0
  Product1 : Product  OutDataType=sfix(16)  OutScaling=2^0  RndMeth=Zero
  W_kW : Constant  Value=single(1000)  OutDataType=sfix(16)  OutScaling=2^0
  Profile_Data : Outport  OutDataType=sfix(16)  OutScaling=2^0
  wires:
  loop_time/1 -> Lookup Table/1
  W_kW/1 -> Product1/2
  Lookup Table/1 -> Product1/1
  Product1/1 -> Profile_Data/1

== system HIL_Testing_SW/LionsHeart/FeaturePresentation/Down_to_Business/DriveProfile_ModeControl/Drive_Profile/CD/Drive_3 ==
  loop_time : Inport  OutDataType=sfix(16)  OutScaling=2^0
  Enable : EnablePort
  Lookup Table : Lookup  InputValues=Drive_3(:,1)  Table=Drive_3(:,2)  OutDataType=fixdt(1, 16)  OutScaling=2^0
  Product1 : Product  OutDataType=sfix(16)  OutScaling=2^0  RndMeth=Zero
  W_kW : Constant  Value=single(1000)  OutDataType=sfix(16)  OutScaling=2^0
  Profile_Data : Outport  OutDataType=sfix(16)  OutScaling=2^0
  wires:
  Product1/1 -> Profile_Data/1
  Lookup Table/1 -> Product1/1
  W_kW/1 -> Product1/2
  loop_time/1 -> Lookup Table/1

== system HIL_Testing_SW/LionsHeart/FeaturePresentation/Down_to_Business/DriveProfile_ModeControl/Drive_Profile/CD/Drive_30 ==
  loop_time : Inport  OutDataType=sfix(16)  OutScaling=2^0
  Enable : EnablePort
  Lookup Table : Lookup  InputValues=Drive_30(:,1)  Table=Drive_30(:,2)  OutDataType=fixdt(1, 16)  OutScaling=2^0
  Product1 : Product  OutDataType=sfix(16)  OutScaling=2^0  RndMeth=Zero
  W_kW : Constant  Value=single(1000)  OutDataType=sfix(16)  OutScaling=2^0
  Profile_Data : Outport  OutDataType=sfix(16)  OutScaling=2^0
  wires:
  Product1/1 -> Profile_Data/1
  Lookup Table/1 -> Product1/1
  W_kW/1 -> Product1/2
  loop_time/1 -> Lookup Table/1

== system HIL_Testing_SW/LionsHeart/FeaturePresentation/Down_to_Business/DriveProfile_ModeControl/Drive_Profile/CD/Drive_31 ==
  loop_time : Inport  OutDataType=sfix(16)  OutScaling=2^0
  Enable : EnablePort
  Lookup Table : Lookup  InputValues=Drive_31(:,1)  Table=Drive_31(:,2)  OutDataType=fixdt(1, 16)  OutScaling=2^0
  Product1 : Product  OutDataType=sfix(16)  OutScaling=2^0  RndMeth=Zero
  W_kW : Constant  Value=single(1000)  OutDataType=sfix(16)  OutScaling=2^0
  Profile_Data : Outport  OutDataType=sfix(16)  OutScaling=2^0
  wires:
  loop_time/1 -> Lookup Table/1
  W_kW/1 -> Product1/2
  Lookup Table/1 -> Product1/1
  Product1/1 -> Profile_Data/1

== system HIL_Testing_SW/LionsHeart/FeaturePresentation/Down_to_Business/DriveProfile_ModeControl/Drive_Profile/CD/Drive_32 ==
  loop_time : Inport  OutDataType=sfix(16)  OutScaling=2^0
  Enable : EnablePort
  Lookup Table : Lookup  InputValues=Drive_32(:,1)  Table=Drive_32(:,2)  OutDataType=fixdt(1, 16)  OutScaling=2^0
  Product1 : Product  OutDataType=sfix(16)  OutScaling=2^0  RndMeth=Zero
  W_kW : Constant  Value=single(1000)  OutDataType=sfix(16)  OutScaling=2^0
  Profile_Data : Outport  OutDataType=sfix(16)  OutScaling=2^0
  wires:
  Product1/1 -> Profile_Data/1
  Lookup Table/1 -> Product1/1
  W_kW/1 -> Product1/2
  loop_time/1 -> Lookup Table/1

== system HIL_Testing_SW/LionsHeart/FeaturePresentation/Down_to_Business/DriveProfile_ModeControl/Drive_Profile/CD/Drive_33 ==
  loop_time : Inport  OutDataType=sfix(16)  OutScaling=2^0
  Enable : EnablePort
  Lookup Table : Lookup  InputValues=Drive_33(:,1)  Table=Drive_33(:,2)  OutDataType=fixdt(1, 16)  OutScaling=2^0
  Product1 : Product  OutDataType=sfix(16)  OutScaling=2^0  RndMeth=Zero
  W_kW : Constant  Value=single(1000)  OutDataType=sfix(16)  OutScaling=2^0
  Profile_Data : Outport  OutDataType=sfix(16)  OutScaling=2^0
  wires:
  loop_time/1 -> Lookup Table/1
  W_kW/1 -> Product1/2
  Lookup Table/1 -> Product1/1
  Product1/1 -> Profile_Data/1

== system HIL_Testing_SW/LionsHeart/FeaturePresentation/Down_to_Business/DriveProfile_ModeControl/Drive_Profile/CD/Drive_34 ==
  loop_time : Inport  OutDataType=sfix(16)  OutScaling=2^0
  Enable : EnablePort
  Lookup Table : Lookup  InputValues=Drive_34(:,1)  Table=Drive_34(:,2)  OutDataType=fixdt(1, 16)  OutScaling=2^0
  Product1 : Product  OutDataType=sfix(16)  OutScaling=2^0  RndMeth=Zero
  W_kW : Constant  Value=single(1000)  OutDataType=sfix(16)  OutScaling=2^0
  Profile_Data : Outport  OutDataType=sfix(16)  OutScaling=2^0
  wires:
  Product1/1 -> Profile_Data/1
  Lookup Table/1 -> Product1/1
  W_kW/1 -> Product1/2
  loop_time/1 -> Lookup Table/1

== system HIL_Testing_SW/LionsHeart/FeaturePresentation/Down_to_Business/DriveProfile_ModeControl/Drive_Profile/CD/Drive_35 ==
  loop_time : Inport  OutDataType=sfix(16)  OutScaling=2^0
  Enable : EnablePort
  Lookup Table : Lookup  InputValues=Drive_35(:,1)  Table=Drive_35(:,2)  OutDataType=fixdt(1, 16)  OutScaling=2^0
  Product1 : Product  OutDataType=sfix(16)  OutScaling=2^0  RndMeth=Zero
  W_kW : Constant  Value=single(1000)  OutDataType=sfix(16)  OutScaling=2^0
  Profile_Data : Outport  OutDataType=sfix(16)  OutScaling=2^0
  wires:
  loop_time/1 -> Lookup Table/1
  W_kW/1 -> Product1/2
  Lookup Table/1 -> Product1/1
  Product1/1 -> Profile_Data/1

== system HIL_Testing_SW/LionsHeart/FeaturePresentation/Down_to_Business/DriveProfile_ModeControl/Drive_Profile/CD/Drive_36 ==
  loop_time : Inport  OutDataType=sfix(16)  OutScaling=2^0
  Enable : EnablePort
  Lookup Table : Lookup  InputValues=Drive_36(:,1)  Table=Drive_36(:,2)  OutDataType=fixdt(1, 16)  OutScaling=2^0
  Product1 : Product  OutDataType=sfix(16)  OutScaling=2^0  RndMeth=Zero
  W_kW : Constant  Value=single(1000)  OutDataType=sfix(16)  OutScaling=2^0
  Profile_Data : Outport  OutDataType=sfix(16)  OutScaling=2^0
  wires:
  Product1/1 -> Profile_Data/1
  Lookup Table/1 -> Product1/1
  W_kW/1 -> Product1/2
  loop_time/1 -> Lookup Table/1

== system HIL_Testing_SW/LionsHeart/FeaturePresentation/Down_to_Business/DriveProfile_ModeControl/Drive_Profile/CD/Drive_37 ==
  loop_time : Inport  OutDataType=sfix(16)  OutScaling=2^0
  Enable : EnablePort
  Lookup Table : Lookup  InputValues=Drive_37(:,1)  Table=Drive_37(:,2)  OutDataType=fixdt(1, 16)  OutScaling=2^0
  Product1 : Product  OutDataType=sfix(16)  OutScaling=2^0  RndMeth=Zero
  W_kW : Constant  Value=single(1000)  OutDataType=sfix(16)  OutScaling=2^0
  Profile_Data : Outport  OutDataType=sfix(16)  OutScaling=2^0
  wires:
  loop_time/1 -> Lookup Table/1
  W_kW/1 -> Product1/2
  Lookup Table/1 -> Product1/1
  Product1/1 -> Profile_Data/1

== system HIL_Testing_SW/LionsHeart/FeaturePresentation/Down_to_Business/DriveProfile_ModeControl/Drive_Profile/CD/Drive_38 ==
  loop_time : Inport  OutDataType=sfix(16)  OutScaling=2^0
  Enable : EnablePort
  Lookup Table : Lookup  InputValues=Drive_38(:,1)  Table=Drive_38(:,2)  OutDataType=fixdt(1, 16)  OutScaling=2^0
  Product1 : Product  OutDataType=sfix(16)  OutScaling=2^0  RndMeth=Zero
  W_kW : Constant  Value=single(1000)  OutDataType=sfix(16)  OutScaling=2^0
  Profile_Data : Outport  OutDataType=sfix(16)  OutScaling=2^0
  wires:
  Product1/1 -> Profile_Data/1
  Lookup Table/1 -> Product1/1
  W_kW/1 -> Product1/2
  loop_time/1 -> Lookup Table/1

== system HIL_Testing_SW/LionsHeart/FeaturePresentation/Down_to_Business/DriveProfile_ModeControl/Drive_Profile/CD/Drive_39 ==
  loop_time : Inport  OutDataType=sfix(16)  OutScaling=2^0
  Enable : EnablePort
  Lookup Table : Lookup  InputValues=Drive_39(:,1)  Table=Drive_39(:,2)  OutDataType=fixdt(1, 16)  OutScaling=2^0
  Product1 : Product  OutDataType=sfix(16)  OutScaling=2^0  RndMeth=Zero
  W_kW : Constant  Value=single(1000)  OutDataType=sfix(16)  OutScaling=2^0
  Profile_Data : Outport  OutDataType=sfix(16)  OutScaling=2^0
  wires:
  loop_time/1 -> Lookup Table/1
  W_kW/1 -> Product1/2
  Lookup Table/1 -> Product1/1
  Product1/1 -> Profile_Data/1

== system HIL_Testing_SW/LionsHeart/FeaturePresentation/Down_to_Business/DriveProfile_ModeControl/Drive_Profile/CD/Drive_4 ==
  loop_time : Inport  OutDataType=sfix(16)  OutScaling=2^0
  Enable : EnablePort
  Lookup Table : Lookup  InputValues=Drive_4(:,1)  Table=Drive_4(:,2)  OutDataType=fixdt(1, 16)  OutScaling=2^0
  Product1 : Product  OutDataType=sfix(16)  OutScaling=2^0  RndMeth=Zero
  W_kW : Constant  Value=single(1000)  OutDataType=sfix(16)  OutScaling=2^0
  Profile_Data : Outport  OutDataType=sfix(16)  OutScaling=2^0
  wires:
  Product1/1 -> Profile_Data/1
  Lookup Table/1 -> Product1/1
  W_kW/1 -> Product1/2
  loop_time/1 -> Lookup Table/1

== system HIL_Testing_SW/LionsHeart/FeaturePresentation/Down_to_Business/DriveProfile_ModeControl/Drive_Profile/CD/Drive_40 ==
  loop_time : Inport  OutDataType=sfix(16)  OutScaling=2^0
  Enable : EnablePort
  Lookup Table : Lookup  InputValues=Drive_40(:,1)  Table=Drive_40(:,2)  OutDataType=fixdt(1, 16)  OutScaling=2^0
  Product1 : Product  OutDataType=sfix(16)  OutScaling=2^0  RndMeth=Zero
  W_kW : Constant  Value=single(1000)  OutDataType=sfix(16)  OutScaling=2^0
  Profile_Data : Outport  OutDataType=sfix(16)  OutScaling=2^0
  wires:
  Product1/1 -> Profile_Data/1
  Lookup Table/1 -> Product1/1
  W_kW/1 -> Product1/2
  loop_time/1 -> Lookup Table/1

== system HIL_Testing_SW/LionsHeart/FeaturePresentation/Down_to_Business/DriveProfile_ModeControl/Drive_Profile/CD/Drive_41 ==
  loop_time : Inport  OutDataType=sfix(16)  OutScaling=2^0
  Enable : EnablePort
  Lookup Table : Lookup  InputValues=Drive_41(:,1)  Table=Drive_41(:,2)  OutDataType=fixdt(1, 16)  OutScaling=2^0
  Product1 : Product  OutDataType=sfix(16)  OutScaling=2^0  RndMeth=Zero
  W_kW : Constant  Value=single(1000)  OutDataType=sfix(16)  OutScaling=2^0
  Profile_Data : Outport  OutDataType=sfix(16)  OutScaling=2^0
  wires:
  loop_time/1 -> Lookup Table/1
  W_kW/1 -> Product1/2
  Lookup Table/1 -> Product1/1
  Product1/1 -> Profile_Data/1

== system HIL_Testing_SW/LionsHeart/FeaturePresentation/Down_to_Business/DriveProfile_ModeControl/Drive_Profile/CD/Drive_42 ==
  loop_time : Inport  OutDataType=sfix(16)  OutScaling=2^0
  Enable : EnablePort
  Lookup Table : Lookup  InputValues=Drive_42(:,1)  Table=Drive_42(:,2)  OutDataType=fixdt(1, 16)  OutScaling=2^0
  Product1 : Product  OutDataType=sfix(16)  OutScaling=2^0  RndMeth=Zero
  W_kW : Constant  Value=single(1000)  OutDataType=sfix(16)  OutScaling=2^0
  Profile_Data : Outport  OutDataType=sfix(16)  OutScaling=2^0
  wires:
  Product1/1 -> Profile_Data/1
  Lookup Table/1 -> Product1/1
  W_kW/1 -> Product1/2
  loop_time/1 -> Lookup Table/1

== system HIL_Testing_SW/LionsHeart/FeaturePresentation/Down_to_Business/DriveProfile_ModeControl/Drive_Profile/CD/Drive_43 ==
  loop_time : Inport  OutDataType=sfix(16)  OutScaling=2^0
  Enable : EnablePort
  Lookup Table : Lookup  InputValues=Drive_43(:,1)  Table=Drive_43(:,2)  OutDataType=fixdt(1, 16)  OutScaling=2^0
  Product1 : Product  OutDataType=sfix(16)  OutScaling=2^0  RndMeth=Zero
  W_kW : Constant  Value=single(1000)  OutDataType=sfix(16)  OutScaling=2^0
  Profile_Data : Outport  OutDataType=sfix(16)  OutScaling=2^0
  wires:
  loop_time/1 -> Lookup Table/1
  W_kW/1 -> Product1/2
  Lookup Table/1 -> Product1/1
  Product1/1 -> Profile_Data/1

== system HIL_Testing_SW/LionsHeart/FeaturePresentation/Down_to_Business/DriveProfile_ModeControl/Drive_Profile/CD/Drive_44 ==
  loop_time : Inport  OutDataType=sfix(16)  OutScaling=2^0
  Enable : EnablePort
  Lookup Table : Lookup  InputValues=Drive_44(:,1)  Table=Drive_44(:,2)  OutDataType=fixdt(1, 16)  OutScaling=2^0
  Product1 : Product  OutDataType=sfix(16)  OutScaling=2^0  RndMeth=Zero
  W_kW : Constant  Value=single(1000)  OutDataType=sfix(16)  OutScaling=2^0
  Profile_Data : Outport  OutDataType=sfix(16)  OutScaling=2^0
  wires:
  Product1/1 -> Profile_Data/1
  Lookup Table/1 -> Product1/1
  W_kW/1 -> Product1/2
  loop_time/1 -> Lookup Table/1

== system HIL_Testing_SW/LionsHeart/FeaturePresentation/Down_to_Business/DriveProfile_ModeControl/Drive_Profile/CD/Drive_45 ==
  loop_time : Inport  OutDataType=sfix(16)  OutScaling=2^0
  Enable : EnablePort
  Lookup Table : Lookup  InputValues=Drive_45(:,1)  Table=Drive_45(:,2)  OutDataType=fixdt(1, 16)  OutScaling=2^0
  Product1 : Product  OutDataType=sfix(16)  OutScaling=2^0  RndMeth=Zero
  W_kW : Constant  Value=single(1000)  OutDataType=sfix(16)  OutScaling=2^0
  Profile_Data : Outport  OutDataType=sfix(16)  OutScaling=2^0
  wires:
  loop_time/1 -> Lookup Table/1
  W_kW/1 -> Product1/2
  Lookup Table/1 -> Product1/1
  Product1/1 -> Profile_Data/1

== system HIL_Testing_SW/LionsHeart/FeaturePresentation/Down_to_Business/DriveProfile_ModeControl/Drive_Profile/CD/Drive_46 ==
  loop_time : Inport  OutDataType=sfix(16)  OutScaling=2^0
  Enable : EnablePort
  Lookup Table : Lookup  InputValues=Drive_46(:,1)  Table=Drive_46(:,2)  OutDataType=fixdt(1, 16)  OutScaling=2^0
  Product1 : Product  OutDataType=sfix(16)  OutScaling=2^0  RndMeth=Zero
  W_kW : Constant  Value=single(1000)  OutDataType=sfix(16)  OutScaling=2^0
  Profile_Data : Outport  OutDataType=sfix(16)  OutScaling=2^0
  wires:
  Product1/1 -> Profile_Data/1
  Lookup Table/1 -> Product1/1
  W_kW/1 -> Product1/2
  loop_time/1 -> Lookup Table/1

== system HIL_Testing_SW/LionsHeart/FeaturePresentation/Down_to_Business/DriveProfile_ModeControl/Drive_Profile/CD/Drive_47 ==
  loop_time : Inport  OutDataType=sfix(16)  OutScaling=2^0
  Enable : EnablePort
  Lookup Table : Lookup  InputValues=Drive_47(:,1)  Table=Drive_47(:,2)  OutDataType=fixdt(1, 16)  OutScaling=2^0
  Product1 : Product  OutDataType=sfix(16)  OutScaling=2^0  RndMeth=Zero
  W_kW : Constant  Value=single(1000)  OutDataType=sfix(16)  OutScaling=2^0
  Profile_Data : Outport  OutDataType=sfix(16)  OutScaling=2^0
  wires:
  loop_time/1 -> Lookup Table/1
  W_kW/1 -> Product1/2
  Lookup Table/1 -> Product1/1
  Product1/1 -> Profile_Data/1

== system HIL_Testing_SW/LionsHeart/FeaturePresentation/Down_to_Business/DriveProfile_ModeControl/Drive_Profile/CD/Drive_48 ==
  loop_time : Inport  OutDataType=sfix(16)  OutScaling=2^0
  Enable : EnablePort
  Lookup Table : Lookup  InputValues=Drive_48(:,1)  Table=Drive_48(:,2)  OutDataType=fixdt(1, 16)  OutScaling=2^0
  Product1 : Product  OutDataType=sfix(16)  OutScaling=2^0  RndMeth=Zero
  W_kW : Constant  Value=single(1000)  OutDataType=sfix(16)  OutScaling=2^0
  Profile_Data : Outport  OutDataType=sfix(16)  OutScaling=2^0
  wires:
  Product1/1 -> Profile_Data/1
  Lookup Table/1 -> Product1/1
  W_kW/1 -> Product1/2
  loop_time/1 -> Lookup Table/1
